simulink model "dynamicFreeplay"  (R2020b)
settings: Solver=VariableStepAuto  StartTime=0.0  StopTime=10.0  RelTol=1e-3
undefined symbols (not defined in the file): freeplayVector, options, stiffness
libraries: simulink x1
settings Model: Creator=Nicola Fonzi  LastModifiedBy=Nicola Fonzi

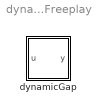
== system dynamicFreeplay ==
  dynamicGap : Subsystem

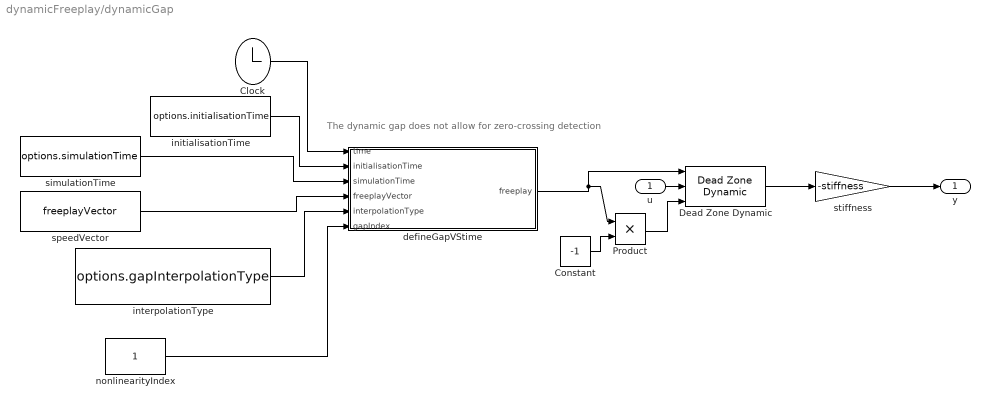
== system dynamicFreeplay/dynamicGap ==
  note: The dynamic gap does not allow for zero-crossing detection
  u : Inport
  Clock : Clock
  Constant : Constant  Value=-1
  Dead Zone Dynamic : simulink/Discontinuities/Dead Zone Dynamic
      settings: SourceProductBaseCode=SL
  Product : Product
  defineGapVStime : MATLAB Function  TreatAsAtomicUnit=on
  initialisationTime : Constant  Value=options.initialisationTime
  interpolationType : Constant  Value=options.gapInterpolationType
  nonlinearityIndex : Constant
  simulationTime : Constant  Value=options.simulationTime
  speedVector : Constant  Value=freeplayVector
  stiffness : Gain  Gain=-stiffness
  y : Outport
  wires:
  u/1 -> Dead Zone Dynamic/2
  Constant/1 -> Product/2
  Product/1 -> Dead Zone Dynamic/3
  interpolationType/1 -> defineGapVStime/5(interpolationType)
  defineGapVStime/1(freeplay) -> Dead Zone Dynamic/1, Product/1
  initialisationTime/1 -> defineGapVStime/2(initialisationTime)
  simulationTime/1 -> defineGapVStime/3(simulationTime)
  speedVector/1 -> defineGapVStime/4(freeplayVector)
  Clock/1 -> defineGapVStime/1(time)
  Dead Zone Dynamic/1 -> stiffness/1
  stiffness/1 -> y/1
  nonlinearityIndex/1 -> defineGapVStime/6(gapIndex)

== matlab function dynamicFreeplay/dynamicGap/defineGapVStime ==
  data: time input; freeplay output; initialisationTime input; simulationTime input; freeplayVector input; interpolationType input; gapIndex input
function freeplay = fcn(time,initialisationTime,simulationTime,freeplayVector,interpolationType,gapIndex)

vectorUsed = freeplayVector{gapIndex};

if time<=initialisationTime
    freeplay = vectorUsed(1);
else
    if interpolationType(gapIndex)==0
        endGap = vectorUsed(end);
        freeplay = interp1(linspace(initialisationTime,simulationTime,length(vectorUsed)+1)...
            ,[vectorUsed, endGap],time,'previous')/2;
    elseif interpolationType(gapIndex)==1
        freeplay = interp1(linspace(initialisationTime,simulationTime,length(vectorUsed))...
            ,vectorUsed,time,"linear")/2;
    else
        freeplay = interp1(linspace(initialisationTime,simulationTime,length(vectorUsed))...
            ,vectorUsed,time,"spline")/2;
    end
end

return
